simulink model "house_heat_start"  (R2018a)
settings: Solver=ode45  StartTime=0.0  StopTime=48  FixedStep=1  RelTol=1e-3  AbsTol=1e-6
PreLoadFcn:
  | load house_heat_data.mat;
values from neighbouring files (symbols this model uses):
  c = 1005.4    [house_heat_data.mat]
  Mdot = 3600    [house_heat_data.mat]
  THeater = 50    [house_heat_data.mat]
Description:
  | Thermal Model of a House
  | 
  | This demo illustrates how you can use Simulink(R) to create the thermal model of
  | a house. This system models the outdoor environment, the thermal
  | characteristics of the house, and the house heating system.
  | 
  | The sldemo_househeat_data.m file initializes data in the model workspace.
  | To make changes, you can edit the model workspace directly or edit the MATLAB(R) file
  | and re-load the model workspace.
  | 
  | To view the model workspace, select View > Model Explorer
  | from the Simulink editor.
  | 
  | Note: Time is given in units of hours
settings Model: ExtModeTrigMode=oneshot  ExtModeArmWhenConnect=off  ExtModeAutoUpdateStatusClock=off  Creator=The MathWorks Inc.  LastModifiedBy=bneiswan
settings SolverCC: AutoScaleAbsTol=off
settings DataIOCC: ExternalInput=[]  InitialState=[]  SaveFormat=Array  SaveOutput=off  SaveTime=off  SignalLoggingName=sldemo_househeat_output
settings OptimizationCC: BlockReduction=off  BooleanDataType=off  ExpressionDepthLimit=2147483647  InitFltsAndDblsToZero=on  LifeSpan=inf  BufferReusableBoundary=off
settings DebuggingCC: SaveWithParameterizedLinksMsg=none  UnderspecifiedInitializationDetection=Classic  MergeDetectMultiDrivingBlocksExec=none  SignalResolutionControl=TryResolveAllWithWarning  MultiTaskDSMMsg=warning  MultiTaskCondExecSysMsg=none  IntegerOverflowMsg=none  ParameterPrecisionLossMsg=none  FcnCallInpInsideContextMsg=warning  BusObjectLabelMismatch=none  AllowSymbolicDim=off  StateNameClashWarn=warning  SFUnexpectedBacktrackingDiag=warning  SFNoUnconditionalDefaultTransitionDiag=warning  SFExecutionAtInitializationDiag=none  IntegerSaturationMsg=none
settings HardwareCC: ProdBitPerPointer=32  ProdBitPerSizeT=32  ProdBitPerPtrDiffT=32  ProdLargestAtomicFloat=None  ProdIntDivRoundTo=Undefined  ProdEndianess=Unspecified  ProdWordSize=32  ProdHWDeviceType=32-bit Generic  TargetUnknown=on
settings ModelReferenceCC: PropagateSignalLabelsOutOfModel=off
settings RTWCC: Description=Generic Real-Time Target
settings CodeAppCC: StateflowObjectComments=on
settings GRTTargetCC: TargetFcnLib=ansi_tfl_tmw.mat  TargetLangStandard=C89/C90 (ANSI)  GeneratePreprocessorConditionals=Disable all  CombineOutputUpdateFcns=off  GRTInterface=on
settings ConfigComp: CovMetricSettings=dw  CovHtmlReporting=on  CovSaveCumulativeToWorkspaceVar=on  CovSaveSingleToWorkspaceVar=on  CovExternalEMLEnable=off  CovSFcnEnable=off

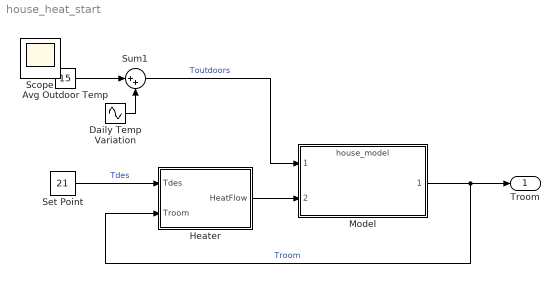
== system house_heat_start ==
  Avg Outdoor Temp : Constant  Value=15
  Daily Temp Variation : Sin  Amplitude=5  Frequency=2*pi/24  SampleTime=0
  Heater : Subsystem
  Model : ModelReference  ModelNameDialog=house_model  ModelReferenceVersion=1.9
  Set Point : Constant  Value=21
  Sum1 : Sum  Inputs=|++  SaturateOnIntegerOverflow=on  InputSameDT=on  OutDataTypeStr=Inherit: Same as first input
  Troom : Outport
  Scope : Scope
  wires:
  Model/1 -> Heater/2(Troom), Troom/1  "Troom"
  Daily Temp Variation/1 -> Sum1/2
  Sum1/1 -> Model/1  "Toutdoors"
  Avg Outdoor Temp/1 -> Sum1/1
  Heater/1(HeatFlow) -> Model/2
  Set Point/1 -> Heater/1(Tdes)  "Tdes"

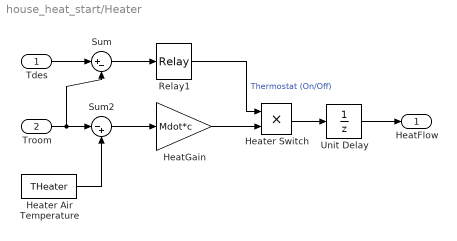
== system house_heat_start/Heater ==
  Tdes : Inport
  Troom : Inport  Port=2
  HeatGain : Gain  Gain=Mdot*c
  Heater Air Temperature : Constant  Value=THeater
  Heater Switch : Product  RndMeth=Zero
  Relay1 : Relay  OnSwitchValue=1  OffSwitchValue=-1
  Sum : Sum  Inputs=|+-  SaturateOnIntegerOverflow=on  InputSameDT=on  OutDataTypeStr=Inherit: Same as first input
  Sum2 : Sum  Inputs=|-+
  Unit Delay : UnitDelay  SampleTime=1/360
  HeatFlow : Outport
  wires:
  Heater Air Temperature/1 -> Sum2/2
  Troom/1 -> Sum2/1, Sum/2
  Sum2/1 -> HeatGain/1
  HeatGain/1 -> Heater Switch/2
  Heater Switch/1 -> Unit Delay/1
  Relay1/1 -> Heater Switch/1  "Thermostat (On/Off)"
  Tdes/1 -> Sum/1
  Sum/1 -> Relay1/1
  Unit Delay/1 -> HeatFlow/1
